simulink model "Operate_lift"  (Simulink 7.4)
settings: Solver=ode3  StartTime=0.0  StopTime=10.0  FixedStep=0.01  RelTol=1e-3
undefined symbols (not defined in the file or in its folder): door_closed, door_open, ElMotor, Elmotor_lib, floor_detected, pos_x
libraries: simulink_extras x5
settings Model: Creator=Maxime Perrotin  LastModifiedBy=Maxime Perrotin
settings DataIOCC: SaveOutput=off  SignalLogging=off  SaveTime=off
settings OptimizationCC: OptimizeModelRefInitCode=on  LifeSpan=1
settings RTWCC: SystemTargetFile=ert.tlc  GenCodeOnly=on  TemplateMakefile=ert_default_tmf  PostCodeGenCommand=packNGo(buildInfo);  Description=Real-Time Workshop Embedded Coder  ProcessScript=ert_make_rtw_hook
settings CodeAppCC: IgnoreCustomStorageClasses=off
settings ERTTargetCC: MultiwordLength=2048  GenerateSampleERTMain=on  SupportContinuousTime=on  ERTCustomFileTemplate=example_file_process.tlc  ConvertIfToSwitch=off

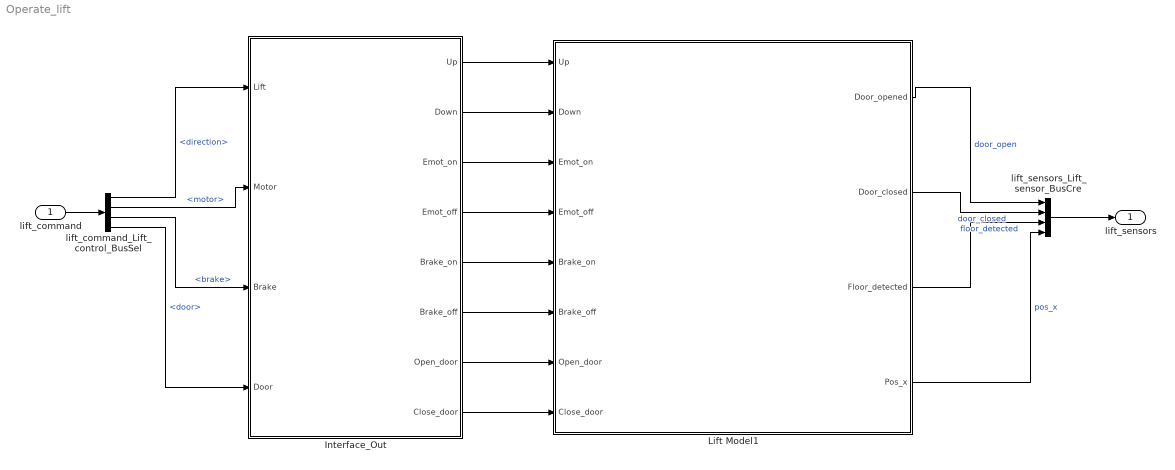
== system Operate_lift ==
  lift_command : Inport  UseBusObject=on  OutDataType=fixdt(1, 16)  OutScaling=2^0
      settings: BusObject=Lift_control
  Interface_Out : Subsystem
  Lift Model1 : Subsystem
  lift_command_Lift_control_BusSel : BusSelector  OutputSignals=direction,motor,brake,door
  lift_sensors_Lift_sensor_BusCre : BusCreator  Inputs=door_open,door_closed,floor_detected,pos_x
      settings: BusObject=Lift_sensor
  lift_sensors : Outport  UseBusObject=on  OutDataType=fixdt(1, 16)  OutScaling=2^0
      settings: BusObject=Lift_sensor
  wires:
  lift_command/1 -> lift_command_Lift_control_BusSel/1
  lift_sensors_Lift_sensor_BusCre/1 -> lift_sensors/1
  Interface_Out/1(Up) -> Lift Model1/1(Up)
  Interface_Out/2(Down) -> Lift Model1/2(Down)
  Interface_Out/3(Emot_on) -> Lift Model1/3(Emot_on)
  Interface_Out/4(Emot_off) -> Lift Model1/4(Emot_off)
  Interface_Out/5(Brake_on) -> Lift Model1/5(Brake_on)
  Interface_Out/6(Brake_off) -> Lift Model1/6(Brake_off)
  Interface_Out/7(Open_door) -> Lift Model1/7(Open_door)
  Interface_Out/8(Close_door) -> Lift Model1/8(Close_door)
  lift_command_Lift_control_BusSel/1 -> Interface_Out/1(Lift)  "<direction>"
  lift_command_Lift_control_BusSel/2 -> Interface_Out/2(Motor)  "<motor>"
  lift_command_Lift_control_BusSel/3 -> Interface_Out/3(Brake)  "<brake>"
  lift_command_Lift_control_BusSel/4 -> Interface_Out/4(Door)  "<door>"
  Lift Model1/1(Door_opened) -> lift_sensors_Lift_sensor_BusCre/1  "door_open"
  Lift Model1/2(Door_closed) -> lift_sensors_Lift_sensor_BusCre/2  "door_closed"
  Lift Model1/3(Floor_detected) -> lift_sensors_Lift_sensor_BusCre/3  "floor_detected"
  Lift Model1/4(Pos_x) -> lift_sensors_Lift_sensor_BusCre/4  "pos_x"

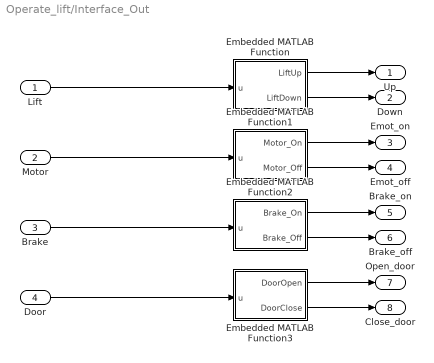
== system Operate_lift/Interface_Out ==
  Lift : Inport
  Motor : Inport  Port=2
  Brake : Inport  Port=3
  Door : Inport  Port=4
  Embedded MATLAB Function : Stateflow chart  TreatAsAtomicUnit=on
  Embedded MATLAB Function1 : Stateflow chart  TreatAsAtomicUnit=on
  Embedded MATLAB Function2 : Stateflow chart  TreatAsAtomicUnit=on
  Embedded MATLAB Function3 : Stateflow chart  TreatAsAtomicUnit=on
  Up : Outport
  Down : Outport  Port=2
  Emot_on : Outport  Port=3
  Emot_off : Outport  Port=4
  Brake_on : Outport  Port=5
  Brake_off : Outport  Port=6
  Open_door : Outport  Port=7
  Close_door : Outport  Port=8
  wires:
  Embedded MATLAB Function3/2(DoorClose) -> Close_door/1
  Embedded MATLAB Function3/1(DoorOpen) -> Open_door/1
  Embedded MATLAB Function2/2(Brake_Off) -> Brake_off/1
  Embedded MATLAB Function2/1(Brake_On) -> Brake_on/1
  Embedded MATLAB Function1/2(Motor_Off) -> Emot_off/1
  Embedded MATLAB Function1/1(Motor_On) -> Emot_on/1
  Embedded MATLAB Function/2(LiftDown) -> Down/1
  Embedded MATLAB Function/1(LiftUp) -> Up/1
  Door/1 -> Embedded MATLAB Function3/1(u)
  Brake/1 -> Embedded MATLAB Function2/1(u)
  Motor/1 -> Embedded MATLAB Function1/1(u)
  Lift/1 -> Embedded MATLAB Function/1(u)

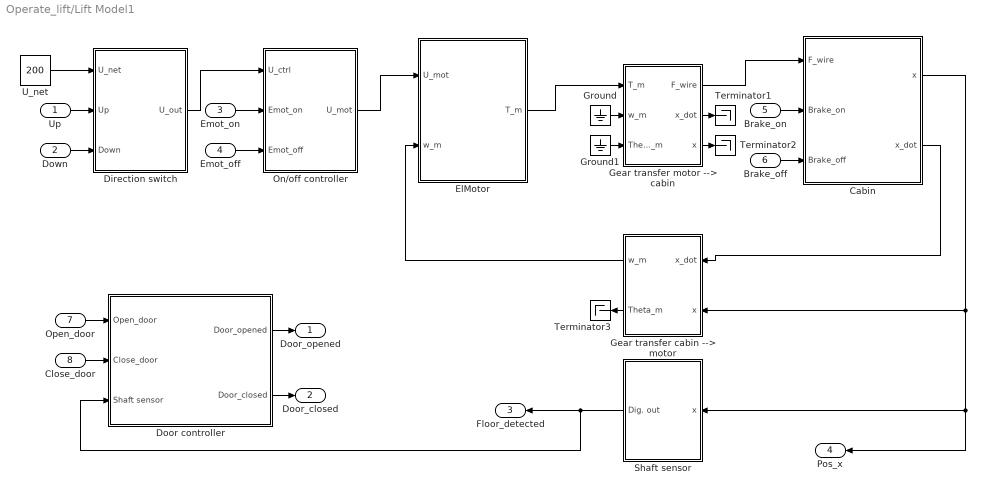
== system Operate_lift/Lift Model1 ==
  Up : Inport
  Down : Inport  Port=2
  Emot_on : Inport  Port=3
  Emot_off : Inport  Port=4
  Brake_on : Inport  Port=5
  Brake_off : Inport  Port=6
  Open_door : Inport  Port=7
  Close_door : Inport  Port=8
  Cabin : Subsystem  Description=Describes the motion of an elevator cabin, with constant mass, influenced by the force in the wire and gravitaion
  Direction switch : Subsystem
  Door controller : Subsystem
  ElMotor : Subsystem  AncestorBlock=Elmotor_lib/ElMotor
  Gear transfer cabin --> motor : Subsystem
  "Gear transfer motor --> cabin " : Subsystem
  Ground : Ground
  Ground1 : Ground
  On/off controller : Subsystem
  Shaft sensor : Subsystem
  Terminator1 : Terminator
  Terminator2 : Terminator
  Terminator3 : Terminator
  U_net : Constant  Value=200
  Door_opened : Outport
  Door_closed : Outport  Port=2
  Floor_detected : Outport  Port=3
  Pos_x : Outport  Port=4
  wires:
  Cabin/1(x) -> Gear transfer cabin --> motor/2(x), Shaft sensor/1(x), Pos_x/1
  Cabin/2(x_dot) -> Gear transfer cabin --> motor/1(x_dot)
  "Gear transfer motor --> cabin "/1(F_wire) -> Cabin/1(F_wire)
  U_net/1 -> Direction switch/1(U_net)
  Direction switch/1(U_out) -> On/off controller/1(U_ctrl)
  On/off controller/1(U_mot) -> ElMotor/1(U_mot)
  ElMotor/1(T_m) -> "Gear transfer motor --> cabin "/1(T_m)
  "Gear transfer motor --> cabin "/2(x_dot) -> Terminator1/1
  "Gear transfer motor --> cabin "/3(x) -> Terminator2/1
  Ground/1 -> "Gear transfer motor --> cabin "/2(w_m)
  Ground1/1 -> "Gear transfer motor --> cabin "/3(Theta_m)
  Shaft sensor/1(Dig. out) -> Door controller/3(Shaft sensor), Floor_detected/1
  Brake_on/1 -> Cabin/2(Brake_on)
  Up/1 -> Direction switch/2(Up)
  Emot_on/1 -> On/off controller/2(Emot_on)
  Down/1 -> Direction switch/3(Down)
  Emot_off/1 -> On/off controller/3(Emot_off)
  Gear transfer cabin --> motor/2(Theta_m) -> Terminator3/1
  Open_door/1 -> Door controller/1(Open_door)
  Door controller/1(Door_opened) -> Door_opened/1
  Close_door/1 -> Door controller/2(Close_door)
  Door controller/2(Door_closed) -> Door_closed/1
  Brake_off/1 -> Cabin/3(Brake_off)
  Gear transfer cabin --> motor/1(w_m) -> ElMotor/2(w_m)

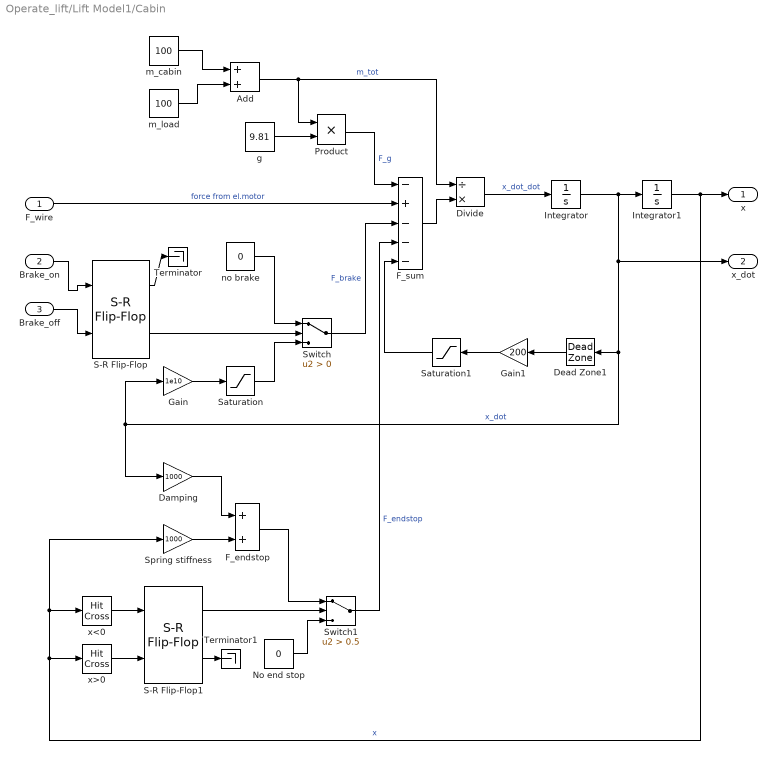
== system Operate_lift/Lift Model1/Cabin ==
  F_wire : Inport
  Brake_on : Inport  Port=2
  Brake_off : Inport  Port=3
  Add : Sum
  Damping : Gain  Gain=1000
  Dead Zone1 : DeadZone  LowerValue=-2  UpperValue=3  SaturateOnIntegerOverflow=on
  Divide : Product  Inputs=/*
  F_endstop : Sum
  F_sum : Sum  Inputs=-+---
  Gain : Gain  Gain=1e10
  Gain1 : Gain  Gain=200
  Integrator : Integrator
  Integrator1 : Integrator  InitialCondition=70
  No end stop : Constant  Value=0
  Product : Product  RndMeth=Zero
  S-R Flip-Flop : simulink_extras/Flip Flops/S-R Flip-Flop  SystemSampleTime=-1  initial_condition=0
  S-R Flip-Flop1 : simulink_extras/Flip Flops/S-R Flip-Flop  SystemSampleTime=-1  initial_condition=0
  Saturation : Saturate  UpperLimit=1e4  LowerLimit=-1e4
  Saturation1 : Saturate  UpperLimit=1e4  LowerLimit=-1e4
  Spring stiffness : Gain  Gain=1000
  Switch : Switch  Criteria=u2 > Threshold
  Switch1 : Switch  Criteria=u2 > Threshold  Threshold=0.5
  Terminator : Terminator
  Terminator1 : Terminator
  g : Constant  Value=9.81
  m_cabin : Constant  Value=100
  m_load : Constant  Value=100
  no brake : Constant  Value=0
  x<0 : HitCross  HitCrossingDirection=falling
  x>0 : HitCross  HitCrossingDirection=rising
  x : Outport
  x_dot : Outport  Port=2
  wires:
  m_cabin/1 -> Add/1
  m_load/1 -> Add/2
  Brake_off/1 -> S-R Flip-Flop/2
  g/1 -> Product/2
  Add/1 -> Product/1, Divide/1  "m_tot"
  Integrator/1 -> Integrator1/1, x_dot/1, Gain/1, Damping/1, Dead Zone1/1  "x_dot"
  Integrator1/1 -> x/1, Spring stiffness/1, x<0/1, x>0/1  "x"
  Divide/1 -> Integrator/1  "x_dot_dot"
  F_wire/1 -> F_sum/2  "force from el.motor"
  Product/1 -> F_sum/1  "F_g"
  S-R Flip-Flop/1 -> Terminator/1
  S-R Flip-Flop/2 -> Switch/2
  Gain/1 -> Saturation/1
  Saturation/1 -> Switch/3
  Switch/1 -> F_sum/3  "F_brake"
  F_sum/1 -> Divide/2
  Damping/1 -> F_endstop/1
  Spring stiffness/1 -> F_endstop/2
  No end stop/1 -> Switch1/3
  Switch1/1 -> F_sum/4  "F_endstop"
  x<0/1 -> S-R Flip-Flop1/1
  S-R Flip-Flop1/1 -> Switch1/2
  S-R Flip-Flop1/2 -> Terminator1/1
  F_endstop/1 -> Switch1/1
  x>0/1 -> S-R Flip-Flop1/2
  no brake/1 -> Switch/1
  Brake_on/1 -> S-R Flip-Flop/1
  Gain1/1 -> Saturation1/1
  Saturation1/1 -> F_sum/5
  Dead Zone1/1 -> Gain1/1

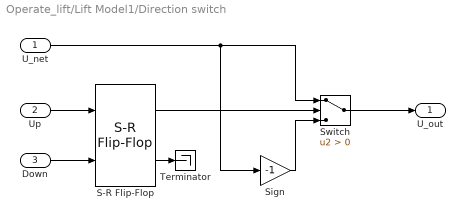
== system Operate_lift/Lift Model1/Direction switch ==
  U_net : Inport
  Up : Inport  Port=2
  Down : Inport  Port=3
  S-R Flip-Flop : simulink_extras/Flip Flops/S-R Flip-Flop  SystemSampleTime=-1  initial_condition=0
  Sign : Gain  Gain=-1
  Switch : Switch  Criteria=u2 > Threshold
  Terminator : Terminator
  U_out : Outport
  wires:
  Up/1 -> S-R Flip-Flop/1
  Down/1 -> S-R Flip-Flop/2
  S-R Flip-Flop/2 -> Terminator/1
  S-R Flip-Flop/1 -> Switch/2
  U_net/1 -> Switch/1, Sign/1
  Sign/1 -> Switch/3
  Switch/1 -> U_out/1

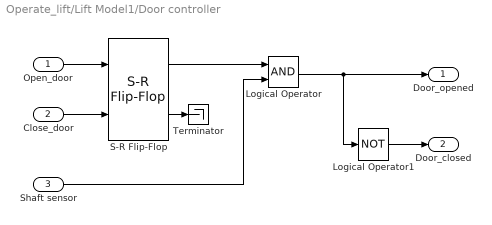
== system Operate_lift/Lift Model1/Door controller ==
  Open_door : Inport
  Close_door : Inport  Port=2
  Shaft sensor : Inport  Port=3
  Logical Operator : Logic  AllPortsSameDT=off  OutDataTypeMode=boolean  OutDataTypeStr=boolean
  Logical Operator1 : Logic  Operator=NOT  AllPortsSameDT=off  OutDataTypeMode=boolean  OutDataTypeStr=boolean
  S-R Flip-Flop : simulink_extras/Flip Flops/S-R Flip-Flop  SystemSampleTime=-1  initial_condition=0
  Terminator : Terminator
  Door_opened : Outport
  Door_closed : Outport  Port=2
  wires:
  Open_door/1 -> S-R Flip-Flop/1
  Close_door/1 -> S-R Flip-Flop/2
  S-R Flip-Flop/2 -> Terminator/1
  Logical Operator/1 -> Door_opened/1, Logical Operator1/1
  Logical Operator1/1 -> Door_closed/1
  S-R Flip-Flop/1 -> Logical Operator/1
  Shaft sensor/1 -> Logical Operator/2

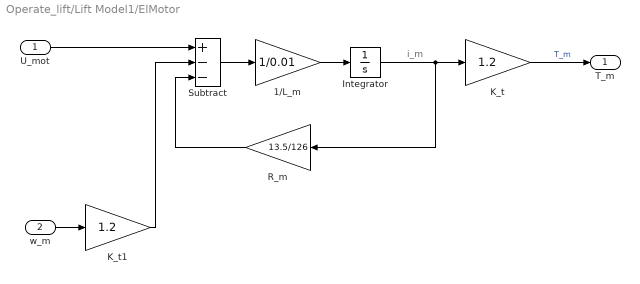
== system Operate_lift/Lift Model1/ElMotor ==
  note: i_m
  U_mot : Inport
  w_m : Inport  Port=2
  1/L_m : Gain  Gain=1/0.01
  Integrator : Integrator
  K_t : Gain  Gain=1.2
  K_t1 : Gain  Gain=1.2
  R_m : Gain  Gain=13.5/126
  Subtract : Sum  Inputs=+--
  T_m : Outport
  wires:
  1/L_m/1 -> Integrator/1
  R_m/1 -> Subtract/3
  K_t1/1 -> Subtract/2
  K_t/1 -> T_m/1  "T_m"
  Subtract/1 -> 1/L_m/1
  Integrator/1 -> K_t/1, R_m/1
  U_mot/1 -> Subtract/1
  w_m/1 -> K_t1/1

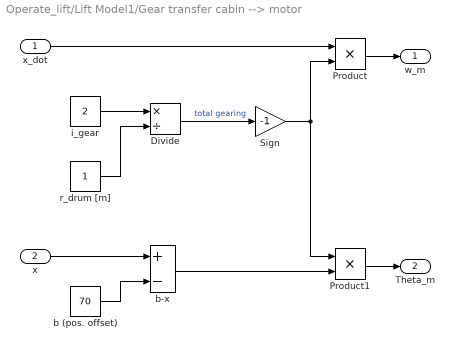
== system Operate_lift/Lift Model1/Gear transfer cabin --> motor ==
  x_dot : Inport
  x : Inport  Port=2
  Divide : Product  Inputs=*/
  Product : Product  RndMeth=Zero
  Product1 : Product  RndMeth=Zero
  Sign : Gain  Gain=-1
  b (pos. offset) : Constant  Value=70
  b-x : Sum  Inputs=+-
  i_gear : Constant  Value=2
  r_drum [m] : Constant
  w_m : Outport
  Theta_m : Outport  Port=2
  wires:
  Product/1 -> w_m/1
  r_drum [m]/1 -> Divide/2
  i_gear/1 -> Divide/1
  x_dot/1 -> Product/1
  Divide/1 -> Sign/1  "total gearing"
  Sign/1 -> Product/2, Product1/1
  x/1 -> b-x/1
  b (pos. offset)/1 -> b-x/2
  Product1/1 -> Theta_m/1
  b-x/1 -> Product1/2

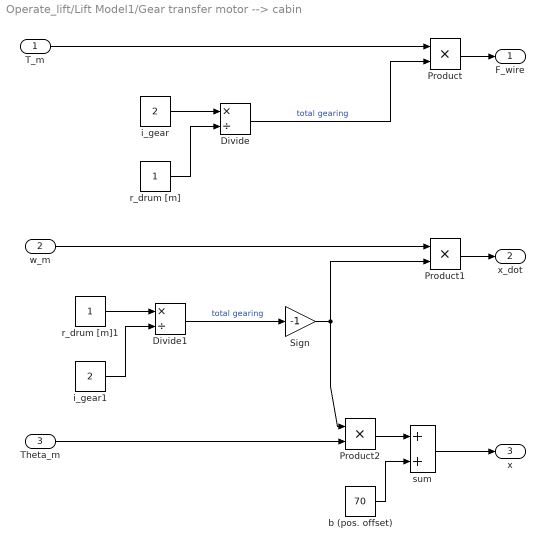
== system Operate_lift/Lift Model1/Gear transfer motor --> cabin  ==
  T_m : Inport
  w_m : Inport  Port=2
  Theta_m : Inport  Port=3
  Divide : Product  Inputs=*/
  Divide1 : Product  Inputs=*/
  Product : Product  RndMeth=Zero
  Product1 : Product  RndMeth=Zero
  Product2 : Product  RndMeth=Zero
  Sign : Gain  Gain=-1
  b (pos. offset) : Constant  Value=70
  i_gear : Constant  Value=2
  i_gear1 : Constant  Value=2
  r_drum [m] : Constant
  r_drum [m]1 : Constant
  sum : Sum
  F_wire : Outport
  x_dot : Outport  Port=2
  x : Outport  Port=3
  wires:
  i_gear/1 -> Divide/1
  r_drum [m]/1 -> Divide/2
  T_m/1 -> Product/1
  Divide/1 -> Product/2  "total gearing"
  Product/1 -> F_wire/1
  Sign/1 -> Product1/2, Product2/1
  Divide1/1 -> Sign/1  "total gearing"
  w_m/1 -> Product1/1
  r_drum [m]1/1 -> Divide1/1
  i_gear1/1 -> Divide1/2
  Product1/1 -> x_dot/1
  Theta_m/1 -> Product2/2
  Product2/1 -> sum/1
  b (pos. offset)/1 -> sum/2
  sum/1 -> x/1

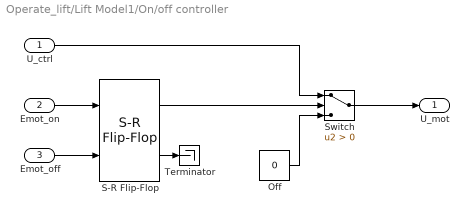
== system Operate_lift/Lift Model1/On/off controller ==
  U_ctrl : Inport
  Emot_on : Inport  Port=2
  Emot_off : Inport  Port=3
  Off : Constant  Value=0
  S-R Flip-Flop : simulink_extras/Flip Flops/S-R Flip-Flop  SystemSampleTime=-1  initial_condition=0
  Switch : Switch  Criteria=u2 > Threshold
  Terminator : Terminator
  U_mot : Outport
  wires:
  Switch/1 -> U_mot/1
  Off/1 -> Switch/3
  U_ctrl/1 -> Switch/1
  S-R Flip-Flop/1 -> Switch/2
  S-R Flip-Flop/2 -> Terminator/1
  Emot_off/1 -> S-R Flip-Flop/2
  Emot_on/1 -> S-R Flip-Flop/1

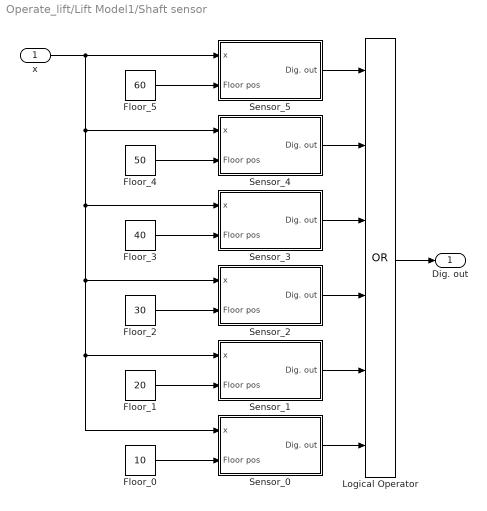
== system Operate_lift/Lift Model1/Shaft sensor ==
  x : Inport
  Floor_0 : Constant  Value=10
  Floor_1 : Constant  Value=20
  Floor_2 : Constant  Value=30
  Floor_3 : Constant  Value=40
  Floor_4 : Constant  Value=50
  Floor_5 : Constant  Value=60
  Logical Operator : Logic  Operator=OR  Inputs=6  AllPortsSameDT=off  OutDataTypeMode=boolean  OutDataTypeStr=boolean
  Sensor_0 : Subsystem
  Sensor_1 : Subsystem
  Sensor_2 : Subsystem
  Sensor_3 : Subsystem
  Sensor_4 : Subsystem
  Sensor_5 : Subsystem
  Dig. out : Outport
  wires:
  Floor_5/1 -> Sensor_5/2(Floor pos)
  x/1 -> Sensor_5/1(x), Sensor_4/1(x), Sensor_3/1(x), Sensor_2/1(x), Sensor_0/1(x), Sensor_1/1(x)
  Floor_0/1 -> Sensor_0/2(Floor pos)
  Floor_1/1 -> Sensor_1/2(Floor pos)
  Floor_2/1 -> Sensor_2/2(Floor pos)
  Floor_3/1 -> Sensor_3/2(Floor pos)
  Floor_4/1 -> Sensor_4/2(Floor pos)
  Sensor_2/1(Dig. out) -> Logical Operator/4
  Sensor_3/1(Dig. out) -> Logical Operator/3
  Sensor_1/1(Dig. out) -> Logical Operator/5
  Sensor_0/1(Dig. out) -> Logical Operator/6
  Sensor_4/1(Dig. out) -> Logical Operator/2
  Sensor_5/1(Dig. out) -> Logical Operator/1
  Logical Operator/1 -> Dig. out/1

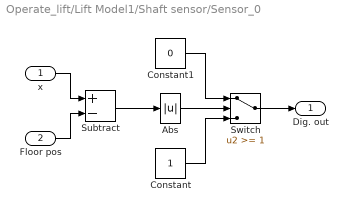
== system Operate_lift/Lift Model1/Shaft sensor/Sensor_0 ==
  x : Inport
  Floor pos : Inport  Port=2
  Abs : Abs
  Constant : Constant  OutDataTypeMode=boolean  OutDataTypeStr=boolean
  Constant1 : Constant  Value=0  OutDataTypeMode=boolean  OutDataTypeStr=boolean
  Subtract : Sum  Inputs=+-
  Switch : Switch  Threshold=1
  Dig. out : Outport
  wires:
  Floor pos/1 -> Subtract/2
  Switch/1 -> Dig. out/1
  x/1 -> Subtract/1
  Constant1/1 -> Switch/1
  Constant/1 -> Switch/3
  Abs/1 -> Switch/2
  Subtract/1 -> Abs/1

== system Operate_lift/Lift Model1/Shaft sensor/Sensor_1 ==
  x : Inport
  Floor pos : Inport  Port=2
  Abs : Abs
  Constant : Constant  OutDataTypeMode=boolean  OutDataTypeStr=boolean
  Constant1 : Constant  Value=0  OutDataTypeMode=boolean  OutDataTypeStr=boolean
  Subtract : Sum  Inputs=+-
  Switch : Switch  Threshold=1
  Dig. out : Outport
  wires:
  Subtract/1 -> Abs/1
  Abs/1 -> Switch/2
  Constant/1 -> Switch/3
  Constant1/1 -> Switch/1
  x/1 -> Subtract/1
  Switch/1 -> Dig. out/1
  Floor pos/1 -> Subtract/2

== system Operate_lift/Lift Model1/Shaft sensor/Sensor_2 ==
  x : Inport
  Floor pos : Inport  Port=2
  Abs : Abs
  Constant : Constant  OutDataTypeMode=boolean  OutDataTypeStr=boolean
  Constant1 : Constant  Value=0  OutDataTypeMode=boolean  OutDataTypeStr=boolean
  Subtract : Sum  Inputs=+-
  Switch : Switch  Threshold=1
  Dig. out : Outport
  wires:
  Floor pos/1 -> Subtract/2
  Switch/1 -> Dig. out/1
  x/1 -> Subtract/1
  Constant1/1 -> Switch/1
  Constant/1 -> Switch/3
  Abs/1 -> Switch/2
  Subtract/1 -> Abs/1

== system Operate_lift/Lift Model1/Shaft sensor/Sensor_3 ==
  x : Inport
  Floor pos : Inport  Port=2
  Abs : Abs
  Constant : Constant  OutDataTypeMode=boolean  OutDataTypeStr=boolean
  Constant1 : Constant  Value=0  OutDataTypeMode=boolean  OutDataTypeStr=boolean
  Subtract : Sum  Inputs=+-
  Switch : Switch  Threshold=1
  Dig. out : Outport
  wires:
  Subtract/1 -> Abs/1
  Abs/1 -> Switch/2
  Constant/1 -> Switch/3
  Constant1/1 -> Switch/1
  x/1 -> Subtract/1
  Switch/1 -> Dig. out/1
  Floor pos/1 -> Subtract/2

== system Operate_lift/Lift Model1/Shaft sensor/Sensor_4 ==
  x : Inport
  Floor pos : Inport  Port=2
  Abs : Abs
  Constant : Constant  OutDataTypeMode=boolean  OutDataTypeStr=boolean
  Constant1 : Constant  Value=0  OutDataTypeMode=boolean  OutDataTypeStr=boolean
  Subtract : Sum  Inputs=+-
  Switch : Switch  Threshold=1
  Dig. out : Outport
  wires:
  Floor pos/1 -> Subtract/2
  Switch/1 -> Dig. out/1
  x/1 -> Subtract/1
  Constant1/1 -> Switch/1
  Constant/1 -> Switch/3
  Abs/1 -> Switch/2
  Subtract/1 -> Abs/1

== system Operate_lift/Lift Model1/Shaft sensor/Sensor_5 ==
  x : Inport
  Floor pos : Inport  Port=2
  Abs : Abs
  Constant : Constant  OutDataTypeMode=boolean  OutDataTypeStr=boolean
  Constant1 : Constant  Value=0  OutDataTypeMode=boolean  OutDataTypeStr=boolean
  Subtract : Sum  Inputs=+-
  Switch : Switch  Threshold=1
  Dig. out : Outport
  wires:
  Subtract/1 -> Abs/1
  Abs/1 -> Switch/2
  Constant/1 -> Switch/3
  Constant1/1 -> Switch/1
  x/1 -> Subtract/1
  Switch/1 -> Dig. out/1
  Floor pos/1 -> Subtract/2

== matlab function Interface_Out/Embedded MATLAB Function ==
  data: u input double; LiftUp output double; LiftDown output double
function [LiftUp,LiftDown]= fcn(u)
%#eml

if u == 0
    LiftUp = false;
    LiftDown = true;
else
    LiftUp = true;
    LiftDown = false;
end

== matlab function Interface_Out/Embedded MATLAB Function1 ==
  data: u input double; Motor_On output double; Motor_Off output double
function [Motor_On,Motor_Off]= fcn(u)
%#eml

if u == 0
    Motor_On = false;
    Motor_Off = true;
else
    Motor_On = true;
    Motor_Off = false;
end

== matlab function Interface_Out/Embedded MATLAB Function2 ==
  data: u input double; Brake_On output double; Brake_Off output double
function [Brake_On,Brake_Off]= fcn(u)
%#eml

if u == 0
    Brake_On = false;
    Brake_Off = true;
else
    Brake_On = true;
    Brake_Off = false;
end

== matlab function Interface_Out/Embedded MATLAB Function3 ==
  data: u input double; DoorOpen output double; DoorClose output double
function [DoorOpen,DoorClose]= fcn(u)
%#eml

if u == 0
    DoorOpen = false;
    DoorClose = true;
else
    DoorOpen = true;
    DoorClose = false;
end
